simulink model "test_motor"  (R2016a)
settings: Solver=VariableStepAuto  StartTime=0.0  StopTime=0.5  RelTol=1e-3
settings Model: Creator=Matias  LastModifiedBy=Matias
settings DataIOCC: SaveFormat=Structure

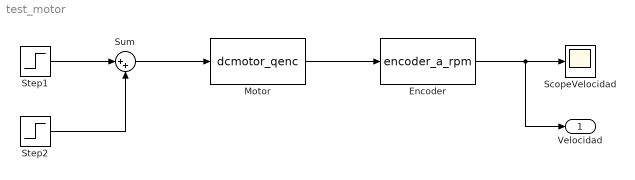
== system test_motor ==
  Encoder : S-Function  FunctionName=encoder_a_rpm  Parameters=0.00001, 0.005,150  SFunctionDeploymentMode=off  EnableBusSupport=off
  Motor : S-Function  FunctionName=dcmotor_qenc  Parameters=150  SFunctionDeploymentMode=off  EnableBusSupport=off
  ScopeVelocidad : Scope
  Step1 : Step  Time=0  After=6  SampleTime=0
  Step2 : Step  Time=0.25  After=6  SampleTime=0
  Sum : Sum  Inputs=|++
  Velocidad : Outport
  wires:
  Motor/1 -> Encoder/1
  Encoder/1 -> Velocidad/1, ScopeVelocidad/1
  Step1/1 -> Sum/1
  Sum/1 -> Motor/1
  Step2/1 -> Sum/2
